simulink model "SIMULINK_U_a_C"  (R2023b)
settings: Solver=FixedStepAuto  StartTime=0.0  StopTime=sim_end_time  FixedStep=fixed_step_size  RelTol=1e-3
undefined symbols (not defined in the file): a, act_end, b, battery_threshold, bb, draw_gif, droneyeeUAV2_NUM, droneyeeUAV3_NUM, droneyeeUAV4_NUM, droneyeeUAV5_NUM, fixed_step_size, k, KD_x, KD_y, kd_z, KDD_x, KDD_y, KI_x, KI_y, ki_z, KII_x, KII_y, KP_x, KP_y, kp_z, KPP_x, KPP_y, lmt, omega, R, sim_end_time, uav10num, uav1num, uav2num, uav3num, uav4num, uav5num, uav6num, uav7num, uav8num, uav9num, UAV_NUM, Vel_Switch_1, Vel_Switch_10, Vel_Switch_11, Vel_Switch_12, Vel_Switch_13, Vel_Switch_14, Vel_Switch_15, Vel_Switch_16, Vel_Switch_17, Vel_Switch_18, Vel_Switch_19, Vel_Switch_2, Vel_Switch_20, Vel_Switch_3, Vel_Switch_4, Vel_Switch_5, Vel_Switch_6, Vel_Switch_7 ... (+11)
libraries: simulink x120, aerolibanimutils x1
(part 4 of 10)

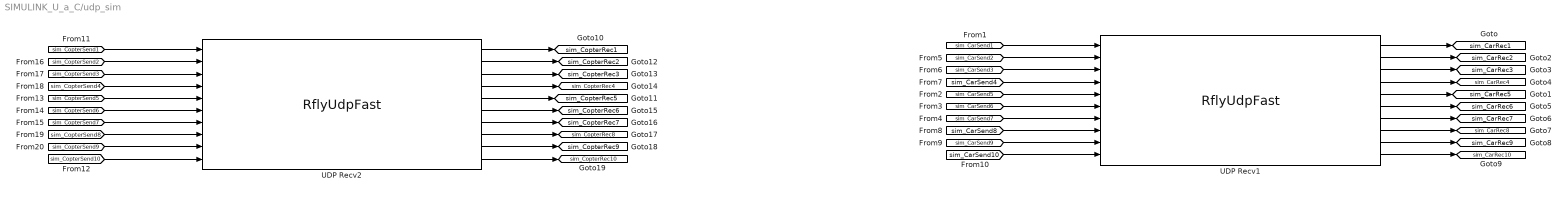
== system SIMULINK_U_a_C/udp_sim ==
  UDP Recv1 : S-Function  FunctionName=RflyUdpFast  Parameters=port,num,modeValue,T,ip  SFunctionDeploymentMode=off  EnableBusSupport=off  mask(UDP Receive){ip=127.0.0.1, port=20100, num=10, mode=UltraSimple Mode, T=1/30, modeValue=0}
      mask prompts: ip "UDP IP Address"; port "UDP Port"; num "vehicle Number"; mode "UDP Mode"; T "Sample Time"
      mask help:
      | This block receives bytes from an UDP/IP connection.
      | The first parameter is the UDP port on the first CopterSim App
      | The second parameter is the total vehicle number
      | The third parameter is the data mode. check the help button for the definition
      mask init:
      | if strcmp(mode,'FullData Mode')
      |     modeValue = 0;
      | elseif strcmp(mode,'SimpleData Mode') 
      |     modeValue = 1;
      | elseif strcmp(mode,'UltraSimple Mode') 
      |     modeValue = 2;
      | else
      |     modeValue = 0;
      | end
      mask Help:
      | UDP mode = 0 (localhost) or 1(broadcast), the 28-D output is defined as:
      | for(int i=0;i<3;i++){
      |     data[0+i]=(double)stl.gpsHome[i];
      |     data[3+i]=(double)stl.AngEular[i];
      |     data[6+i]=(double)stl.localPos[i];
      |     data[9+i]=(double)stl.localVel[i];
      |     data[12+i]=(double)stl.GpsPos[i];
      |     data[15+i]=(double)stl.GpsVel[i];
      | }
      | data[18] = (double)stl.time_boot_ms;
      | data[19] = (double)stl.copterID;
      | data[20] = (double)stl.relative_alt;
      | data[21] = (double)stl.hdg;
      | data[22] = (double)stl.satellites_visible;
      | data[23] = (double)stl.fix_type;
      | data[24] = (double)stl.resrveInit;
      | data[25] = (double)stl.pos_horiz_accuracy;
      | data[26] = (double)stl.pos_vert_accuracy;
      | data[27] = (double)stl.resrveFloat;
      | 
      | UDP mode =  2 (localhost) or 3(broadcast), 4,5 the 12-D output is defined as:
      | 
      | if(iUdpMode==2||iUdpMode==3){
      |     for(int i=0;i<3;i++){
      |         data[i]=(double)st.gpsHome[i];
      |         data[i+3]=(double)st.AngEular[i];
      |         data[i+6]=(double)st.localPos[i];
      |         data[i+9]=(double)st.localVel[i];
      |     }
      | }
      | if(iUdpMode==4||iUdpMode==5){
      |     double GpsHomePos[3];
      |     for(int i=0;i<3;i++){
      |             GpsHomePos[i] = (double)st.gpsHome[i];
      |             data[3+i]=(double)st.localPos[i];
      |             data[6+i]=(double)st.localVel[i];
      |             data[9+i]=(double)st.AngEular[i];
      |     }
      |     double PIR = 3.1415926536;
      |     data[0]=(GpsHomePos[0]*1e-7-40.1540302)/180*PIR*6362000+(double)st.localPos[0];
      |     data[1]=(GpsHomePos[1]*1e-7-116.2593683)/180*PIR*6362000+(double)st.localPos[1];
      |     data[2]=-GpsHomePos[2]*1e-3+(double)st.localPos[2];
      | }
      | 
      | The above structure is
      | struct outHILStateData{ // mavlink data forward from Pixhawk
      |     uint32_t time_boot_ms; //Timestamp of the message
      |     uint32_t copterID;     //Copter ID start from 1
      |     int32_t GpsPos[3];     //Estimated GPS position，lat&long: deg*1e7, alt: m*1e3 and up is positive
      |     int32_t GpsVel[3];     //Estimated GPS velocity, NED, m/s*1e2->cm/s
      |     int32_t gpsHome[3];     //Home GPS position, lat&long: deg*1e7, alt: m*1e3 and up is positive
      |     int32_t relative_alt;  //alt: m*1e3 and up is positive
      |     int32_t hdg;           //Course angle, NED,deg*1000, 0~360
      |     int32_t satellites_visible; //GPS Raw data, sum of satellite
      |     int32_t fix_type;     //GPS Raw data, Fixed type, 3 for fixed (good precision)
      |     int32_t resrveInit;       //Int, reserve for the future use
      |     float AngEular[3];    //Estimated Euler angle, unit: rad/s
      |     float localPos[3];    //Estimated locoal position, NED, unit: m
      |     float localVel[3];    //Estimated locoal velocity, NED, unit: m/s
      |     float pos_horiz_accuracy;   //GPS horizontal accuracy, unit: m
      |     float pos_vert_accuracy; //GPS vertical accuracy, unit: m
      |     float resrveFloat;      //float,reserve for the future use
      | }
      mask TypeOptions mode: FullData Mode | SimpleData Mode | UltraSimple Mode
  UDP Recv2 : S-Function  FunctionName=RflyUdpFast  Parameters=port,num,modeValue,T,ip  SFunctionDeploymentMode=off  EnableBusSupport=off  mask(UDP Receive){ip=127.0.0.1, port=20100, num=10, mode=UltraSimple Mode, T=1/30, modeValue=0}
      mask prompts: ip "UDP IP Address"; port "UDP Port"; num "vehicle Number"; mode "UDP Mode"; T "Sample Time"
      mask help:
      | This block receives bytes from an UDP/IP connection.
      | The first parameter is the UDP port on the first CopterSim App
      | The second parameter is the total vehicle number
      | The third parameter is the data mode. check the help button for the definition
      mask init:
      | if strcmp(mode,'FullData Mode')
      |     modeValue = 0;
      | elseif strcmp(mode,'SimpleData Mode') 
      |     modeValue = 1;
      | elseif strcmp(mode,'UltraSimple Mode') 
      |     modeValue = 2;
      | else
      |     modeValue = 0;
      | end
      mask Help:
      | UDP mode = 0 (localhost) or 1(broadcast), the 28-D output is defined as:
      | for(int i=0;i<3;i++){
      |     data[0+i]=(double)stl.gpsHome[i];
      |     data[3+i]=(double)stl.AngEular[i];
      |     data[6+i]=(double)stl.localPos[i];
      |     data[9+i]=(double)stl.localVel[i];
      |     data[12+i]=(double)stl.GpsPos[i];
      |     data[15+i]=(double)stl.GpsVel[i];
      | }
      | data[18] = (double)stl.time_boot_ms;
      | data[19] = (double)stl.copterID;
      | data[20] = (double)stl.relative_alt;
      | data[21] = (double)stl.hdg;
      | data[22] = (double)stl.satellites_visible;
      | data[23] = (double)stl.fix_type;
      | data[24] = (double)stl.resrveInit;
      | data[25] = (double)stl.pos_horiz_accuracy;
      | data[26] = (double)stl.pos_vert_accuracy;
      | data[27] = (double)stl.resrveFloat;
      | 
      | UDP mode =  2 (localhost) or 3(broadcast), 4,5 the 12-D output is defined as:
      | 
      | if(iUdpMode==2||iUdpMode==3){
      |     for(int i=0;i<3;i++){
      |         data[i]=(double)st.gpsHome[i];
      |         data[i+3]=(double)st.AngEular[i];
      |         data[i+6]=(double)st.localPos[i];
      |         data[i+9]=(double)st.localVel[i];
      |     }
      | }
      | if(iUdpMode==4||iUdpMode==5){
      |     double GpsHomePos[3];
      |     for(int i=0;i<3;i++){
      |             GpsHomePos[i] = (double)st.gpsHome[i];
      |             data[3+i]=(double)st.localPos[i];
      |             data[6+i]=(double)st.localVel[i];
      |             data[9+i]=(double)st.AngEular[i];
      |     }
      |     double PIR = 3.1415926536;
      |     data[0]=(GpsHomePos[0]*1e-7-40.1540302)/180*PIR*6362000+(double)st.localPos[0];
      |     data[1]=(GpsHomePos[1]*1e-7-116.2593683)/180*PIR*6362000+(double)st.localPos[1];
      |     data[2]=-GpsHomePos[2]*1e-3+(double)st.localPos[2];
      | }
      | 
      | The above structure is
      | struct outHILStateData{ // mavlink data forward from Pixhawk
      |     uint32_t time_boot_ms; //Timestamp of the message
      |     uint32_t copterID;     //Copter ID start from 1
      |     int32_t GpsPos[3];     //Estimated GPS position，lat&long: deg*1e7, alt: m*1e3 and up is positive
      |     int32_t GpsVel[3];     //Estimated GPS velocity, NED, m/s*1e2->cm/s
      |     int32_t gpsHome[3];     //Home GPS position, lat&long: deg*1e7, alt: m*1e3 and up is positive
      |     int32_t relative_alt;  //alt: m*1e3 and up is positive
      |     int32_t hdg;           //Course angle, NED,deg*1000, 0~360
      |     int32_t satellites_visible; //GPS Raw data, sum of satellite
      |     int32_t fix_type;     //GPS Raw data, Fixed type, 3 for fixed (good precision)
      |     int32_t resrveInit;       //Int, reserve for the future use
      |     float AngEular[3];    //Estimated Euler angle, unit: rad/s
      |     float localPos[3];    //Estimated locoal position, NED, unit: m
      |     float localVel[3];    //Estimated locoal velocity, NED, unit: m/s
      |     float pos_horiz_accuracy;   //GPS horizontal accuracy, unit: m
      |     float pos_vert_accuracy; //GPS vertical accuracy, unit: m
      |     float resrveFloat;      //float,reserve for the future use
      | }
      mask TypeOptions mode: FullData Mode | SimpleData Mode | UltraSimple Mode
  tag scope: sim_CarRec10=global, sim_CarRec1=global, sim_CarRec2=global, sim_CarRec3=global, sim_CarRec4=global, sim_CarRec5=global, sim_CarRec6=global, sim_CarRec7=global, sim_CarRec8=global, sim_CarRec9=global, sim_CopterRec10=global, sim_CopterRec1=global, sim_CopterRec2=global, sim_CopterRec3=global, sim_CopterRec4=global, sim_CopterRec5=global, sim_CopterRec6=global, sim_CopterRec7=global, sim_CopterRec8=global, sim_CopterRec9=global
  wires:
  UDP Recv1/9 -> [sim_CarRec9]
  UDP Recv1/8 -> [sim_CarRec8]
  [sim_CarSend10] -> UDP Recv1/10
  [sim_CarSend3] -> UDP Recv1/3
  [sim_CarSend5] -> UDP Recv1/5
  [sim_CarSend9] -> UDP Recv1/9
  [sim_CarSend6] -> UDP Recv1/6
  UDP Recv1/1 -> [sim_CarRec1]
  [sim_CarSend8] -> UDP Recv1/8
  UDP Recv1/7 -> [sim_CarRec7]
  UDP Recv1/5 -> [sim_CarRec5]
  UDP Recv1/2 -> [sim_CarRec2]
  [sim_CarSend7] -> UDP Recv1/7
  [sim_CarSend4] -> UDP Recv1/4
  UDP Recv1/4 -> [sim_CarRec4]
  UDP Recv1/10 -> [sim_CarRec10]
  [sim_CarSend2] -> UDP Recv1/2
  UDP Recv1/6 -> [sim_CarRec6]
  [sim_CarSend1] -> UDP Recv1/1
  UDP Recv1/3 -> [sim_CarRec3]
  [sim_CopterSend3] -> UDP Recv2/3
  UDP Recv2/5 -> [sim_CopterRec5]
  UDP Recv2/7 -> [sim_CopterRec7]
  UDP Recv2/6 -> [sim_CopterRec6]
  UDP Recv2/1 -> [sim_CopterRec1]
  [sim_CopterSend7] -> UDP Recv2/7
  [sim_CopterSend2] -> UDP Recv2/2
  [sim_CopterSend10] -> UDP Recv2/10
  UDP Recv2/9 -> [sim_CopterRec9]
  [sim_CopterSend8] -> UDP Recv2/8
  UDP Recv2/2 -> [sim_CopterRec2]
  UDP Recv2/10 -> [sim_CopterRec10]
  UDP Recv2/8 -> [sim_CopterRec8]
  UDP Recv2/3 -> [sim_CopterRec3]
  [sim_CopterSend9] -> UDP Recv2/9
  [sim_CopterSend4] -> UDP Recv2/4
  [sim_CopterSend6] -> UDP Recv2/6
  [sim_CopterSend1] -> UDP Recv2/1
  [sim_CopterSend5] -> UDP Recv2/5
  UDP Recv2/4 -> [sim_CopterRec4]

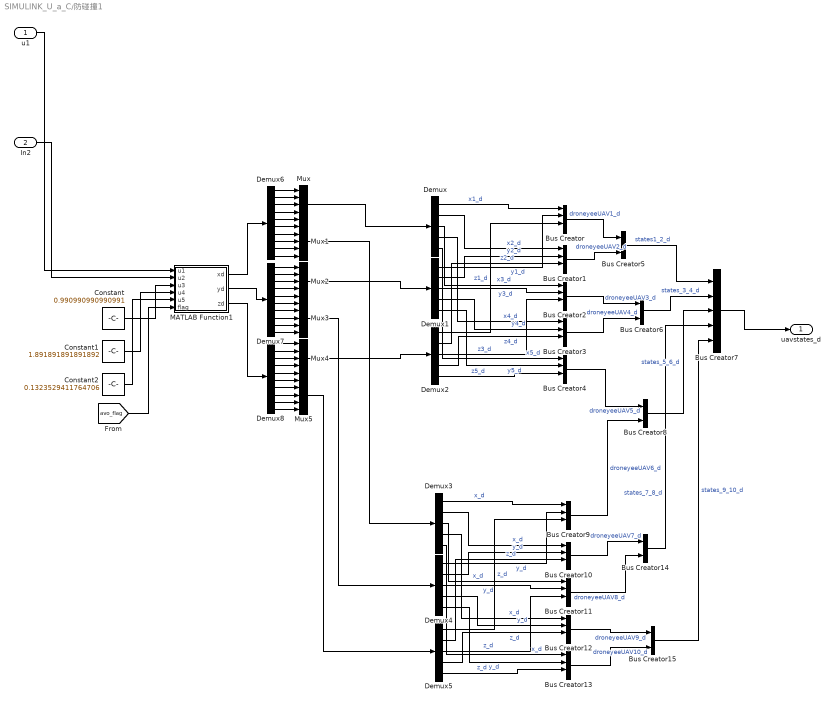
== system SIMULINK_U_a_C/防碰撞1 ==
  u1 : Inport
  In2 : Inport  Port=2
  Bus Creator{,1..4,9..13} (10 alike) : BusCreator  Inputs=4
  Bus Creator{5..6,8,14..15} (5 alike) : BusCreator  Inputs=2
  Bus Creator7 : BusCreator  Inputs=5
  Constant : Constant  Value=0.990990990990991
  Constant1 : Constant  Value=1.891891891891892
  Constant2 : Constant  Value=0.1323529411764706
  Demux{,1..5} (6 alike) : Demux  Outputs=5
  Demux6 : Demux  Outputs=10
  Demux7 : Demux  Outputs=10
  Demux8 : Demux  Outputs=10
  MATLAB Function1 : MATLAB Function
  Mux{,1..5} (6 alike) : Mux  Inputs=5
  uavstates_d : Outport  VectorParamsAs1DForOutWhenUnconnected=off
  wires:
  Bus Creator3/1 -> Bus Creator6/2  "droneyeeUAV4_d"
  Bus Creator1/1 -> Bus Creator5/2  "droneyeeUAV2_d"
  Bus Creator2/1 -> Bus Creator6/1  "droneyeeUAV3_d"
  Demux1/2 -> Bus Creator1/2  "y2_d"
  Bus Creator/1 -> Bus Creator5/1  "droneyeeUAV1_d"
  Bus Creator4/1 -> Bus Creator8/1  "droneyeeUAV5_d"
  Bus Creator6/1 -> Bus Creator7/2  "states_3_4_d"
  Bus Creator5/1 -> Bus Creator7/1  "states1_2_d"
  In2/1 -> MATLAB Function1/2(u2)
  u1/1 -> MATLAB Function1/1(u1)
  Demux2/2 -> Bus Creator1/3  "z2_d"
  Demux2/4 -> Bus Creator3/3  "z4_d"
  Demux/3 -> Bus Creator2/1  "x3_d"
  Demux2/5 -> Bus Creator4/3  "z5_d"
  Demux1/4 -> Bus Creator3/2  "y4_d"
  MATLAB Function1/3(zd) -> Demux8/1
  MATLAB Function1/2(yd) -> Demux7/1
  Demux1/5 -> Bus Creator4/2  "y5_d"
  Demux1/3 -> Bus Creator2/2  "y3_d"
  Demux2/3 -> Bus Creator2/3  "z3_d"
  Demux/4 -> Bus Creator3/1  "x4_d"
  Demux/5 -> Bus Creator4/1  "x5_d"
  Demux/1 -> Bus Creator/1  "x1_d"
  Demux/2 -> Bus Creator1/1  "x2_d"
  Demux1/1 -> Bus Creator/2  "y1_d"
  Demux2/1 -> Bus Creator/3  "z1_d"
  MATLAB Function1/1(xd) -> Demux6/1
  Bus Creator7/1 -> uavstates_d/1
  ? -> Bus Creator/4  "yaw1_d"
  ? -> Bus Creator1/4  "yaw2_d"
  ? -> Bus Creator2/4  "yaw3_d"
  ? -> Bus Creator3/4  "yaw4_d"
  ? -> Bus Creator4/4  "yaw5_d"
  Constant/1 -> MATLAB Function1/3(u3)
  Constant1/1 -> MATLAB Function1/4(u4)
  Constant2/1 -> MATLAB Function1/5(u5)
  ? -> Bus Creator13/4  "yaw_d"
  ? -> Bus Creator11/4  "yaw_d"
  ? -> Bus Creator10/4  "yaw_d"
  ? -> Bus Creator9/4  "yaw_d"
  ? -> Bus Creator12/4  "yaw_d"
  Demux5/2 -> Bus Creator10/3  "z_d"
  Demux3/2 -> Bus Creator10/1  "x_d"
  Demux5/5 -> Bus Creator13/3  "z_d"
  Demux3/4 -> Bus Creator12/1  "x_d"
  Demux3/1 -> Bus Creator9/1  "x_d"
  Demux5/4 -> Bus Creator12/3  "z_d"
  Demux5/1 -> Bus Creator9/3  "z_d"
  Demux5/3 -> Bus Creator11/3  "z_d"
  Demux4/1 -> Bus Creator9/2  "y_d"
  Demux4/3 -> Bus Creator11/2  "y_d"
  Demux3/5 -> Bus Creator13/1  "x_d"
  Demux3/3 -> Bus Creator11/1  "x_d"
  Demux4/4 -> Bus Creator12/2  "y_d"
  Demux4/2 -> Bus Creator10/2  "y_d"
  Demux4/5 -> Bus Creator13/2  "y_d"
  Demux6/1 -> Mux/1
  Demux6/2 -> Mux/2
  Demux6/3 -> Mux/3
  Demux6/4 -> Mux/4
  Demux6/5 -> Mux/5
  Demux6/6 -> Mux1/1
  Demux6/7 -> Mux1/2
  Demux6/8 -> Mux1/3
  Demux6/9 -> Mux1/4
  Demux6/10 -> Mux1/5
  Demux7/6 -> Mux3/1
  Demux7/10 -> Mux3/5
  Demux7/8 -> Mux3/3
  Demux7/4 -> Mux2/4
  Demux7/3 -> Mux2/3
  Demux7/5 -> Mux2/5
  Demux7/7 -> Mux3/2
  Demux7/2 -> Mux2/2
  Demux7/9 -> Mux3/4
  Demux7/1 -> Mux2/1
  Demux8/6 -> Mux5/1
  Demux8/10 -> Mux5/5
  Demux8/8 -> Mux5/3
  Demux8/4 -> Mux4/4
  Demux8/3 -> Mux4/3
  Demux8/5 -> Mux4/5
  Demux8/7 -> Mux5/2
  Demux8/2 -> Mux4/2
  Demux8/9 -> Mux5/4
  Demux8/1 -> Mux4/1
  Mux/1 -> Demux/1
  Mux1/1 -> Demux3/1
  Mux2/1 -> Demux1/1
  Mux3/1 -> Demux4/1
  Mux4/1 -> Demux2/1
  Mux5/1 -> Demux5/1
  [avo_flag] -> MATLAB Function1/6(flag)
  Bus Creator9/1 -> Bus Creator8/2  "droneyeeUAV6_d"
  Bus Creator8/1 -> Bus Creator7/3  "states_5_6_d"
  Bus Creator10/1 -> Bus Creator14/1  "droneyeeUAV7_d"
  Bus Creator11/1 -> Bus Creator14/2  "droneyeeUAV8_d"
  Bus Creator12/1 -> Bus Creator15/1  "droneyeeUAV9_d"
  Bus Creator13/1 -> Bus Creator15/2  "droneyeeUAV10_d"
  Bus Creator14/1 -> Bus Creator7/4  "states_7_8_d"
  Bus Creator15/1 -> Bus Creator7/5  "states_9_10_d"

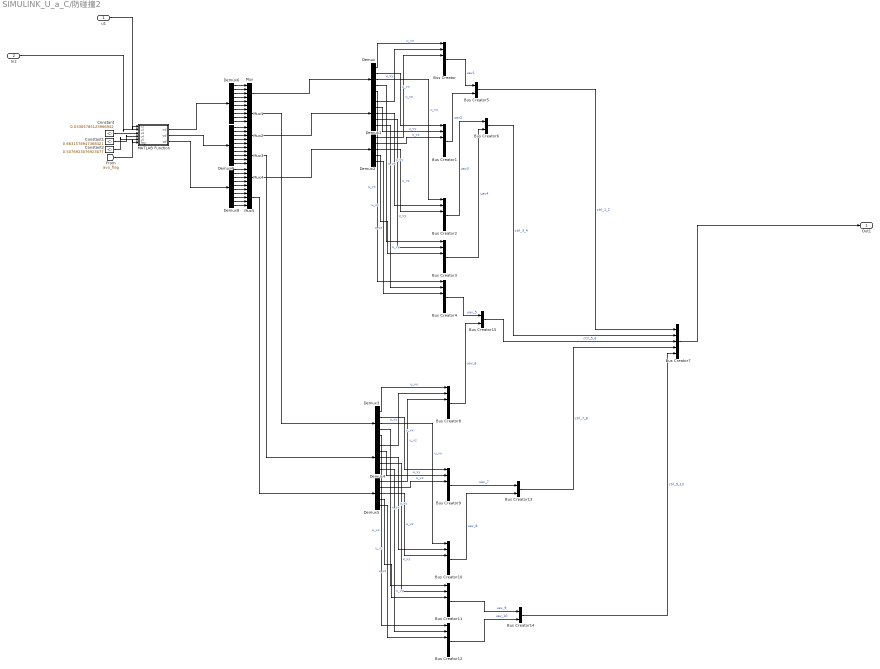
== system SIMULINK_U_a_C/防碰撞2 ==
  u1 : Inport
  In2 : Inport  Port=2
  Bus Creator{,1..4,8..12} (10 alike) : BusCreator  Inputs=6
  Bus Creator{5..6,13..15} (5 alike) : BusCreator  Inputs=2
  Bus Creator7 : BusCreator  Inputs=5
  Constant : Constant  Value=0.03305785123966942
  Constant1 : Constant  Value=0.6631578947368421
  Constant2 : Constant  Value=0.5076923076923077
  Demux{,1..5} (6 alike) : Demux  Outputs=5
  Demux6 : Demux  Outputs=10
  Demux7 : Demux  Outputs=10
  Demux8 : Demux  Outputs=10
  MATLAB Function : MATLAB Function
  Mux{,1..5} (6 alike) : Mux  Inputs=5
  Out1 : Outport  VectorParamsAs1DForOutWhenUnconnected=off
  wires:
  Bus Creator3/1 -> Bus Creator6/2  "uav4"
  Bus Creator1/1 -> Bus Creator5/2  "uav2"
  Bus Creator2/1 -> Bus Creator6/1  "uav3"
  Bus Creator/1 -> Bus Creator5/1  "uav1"
  Bus Creator15/1 -> Bus Creator7/3  "ctrl_5_6"
  Bus Creator6/1 -> Bus Creator7/2  "ctrl_3_4"
  Bus Creator5/1 -> Bus Creator7/1  "ctrl_1_2"
  In2/1 -> MATLAB Function/2(u2)
  u1/1 -> MATLAB Function/1(u1)
  MATLAB Function/3(zd) -> Demux8/1
  MATLAB Function/2(yd) -> Demux7/1
  Demux/1 -> Bus Creator/1  "u_vx"
  Demux1/1 -> Bus Creator/2  "u_vy"
  Demux2/1 -> Bus Creator/3  "u_vz"
  MATLAB Function/1(xd) -> Demux6/1
  Bus Creator7/1 -> Out1/1
  ? -> Bus Creator/4  "u_rate_roll"
  ? -> Bus Creator/5  "u_rate_pitch"
  ? -> Bus Creator/6  "u_rate_yaw"
  ? -> Bus Creator4/6  "u_rate_yaw"
  ? -> Bus Creator4/4  "u_rate_roll"
  Demux2/5 -> Bus Creator4/3  "u_vz"
  Demux/5 -> Bus Creator4/1  "u_vx"
  Demux1/5 -> Bus Creator4/2  "u_vy"
  ? -> Bus Creator4/5  "u_rate_pitch"
  ? -> Bus Creator3/6  "u_rate_yaw"
  ? -> Bus Creator3/4  "u_rate_roll"
  Demux2/4 -> Bus Creator3/3  "u_vz"
  Demux/4 -> Bus Creator3/1  "u_vx"
  Demux1/4 -> Bus Creator3/2  "u_vy"
  ? -> Bus Creator3/5  "u_rate_pitch"
  ? -> Bus Creator2/6  "u_rate_yaw"
  ? -> Bus Creator2/4  "u_rate_roll"
  Demux2/3 -> Bus Creator2/3  "u_vz"
  Demux/3 -> Bus Creator2/1  "u_vx"
  Demux1/3 -> Bus Creator2/2  "u_vy"
  ? -> Bus Creator2/5  "u_rate_pitch"
  ? -> Bus Creator1/6  "u_rate_yaw"
  ? -> Bus Creator1/4  "u_rate_roll"
  Demux2/2 -> Bus Creator1/3  "u_vz"
  Demux/2 -> Bus Creator1/1  "u_vx"
  Demux1/2 -> Bus Creator1/2  "u_vy"
  ? -> Bus Creator1/5  "u_rate_pitch"
  Constant/1 -> MATLAB Function/3(u3)
  Constant1/1 -> MATLAB Function/4(u4)
  Constant2/1 -> MATLAB Function/5(u5)
  Demux3/1 -> Bus Creator8/1  "u_vx"
  Demux5/3 -> Bus Creator10/3  "u_vz"
  Demux4/4 -> Bus Creator11/2  "u_vy"
  ? -> Bus Creator10/4  "u_rate_roll"
  ? -> Bus Creator10/5  "u_rate_pitch"
  ? -> Bus Creator9/5  "u_rate_pitch"
  Demux5/1 -> Bus Creator8/3  "u_vz"
  Demux3/2 -> Bus Creator9/1  "u_vx"
  Demux4/2 -> Bus Creator9/2  "u_vy"
  Demux3/5 -> Bus Creator12/1  "u_vx"
  Bus Creator10/1 -> Bus Creator13/2  "uav_8"
  Demux4/5 -> Bus Creator12/2  "u_vy"
  Demux3/4 -> Bus Creator11/1  "u_vx"
  Demux3/3 -> Bus Creator10/1  "u_vx"
  ? -> Bus Creator10/6  "u_rate_yaw"
  Demux5/4 -> Bus Creator11/3  "u_vz"
  ? -> Bus Creator9/6  "u_rate_yaw"
  Demux5/2 -> Bus Creator9/3  "u_vz"
  Demux4/3 -> Bus Creator10/2  "u_vy"
  ? -> Bus Creator12/5  "u_rate_pitch"
  ? -> Bus Creator9/4  "u_rate_roll"
  ? -> Bus Creator12/6  "u_rate_yaw"
  ? -> Bus Creator8/6  "u_rate_yaw"
  ? -> Bus Creator11/6  "u_rate_yaw"
  ? -> Bus Creator8/4  "u_rate_roll"
  ? -> Bus Creator11/4  "u_rate_roll"
  Bus Creator9/1 -> Bus Creator13/1  "uav_7"
  Bus Creator11/1 -> Bus Creator14/1  "uav_9"
  ? -> Bus Creator8/5  "u_rate_pitch"
  Bus Creator8/1 -> Bus Creator15/2  "uav_6"
  Demux4/1 -> Bus Creator8/2  "u_vy"
  ? -> Bus Creator11/5  "u_rate_pitch"
  ? -> Bus Creator12/4  "u_rate_roll"
  Demux5/5 -> Bus Creator12/3  "u_vz"
  Demux6/4 -> Mux/4
  Demux6/3 -> Mux/3
  Demux6/2 -> Mux/2
  Demux8/7 -> Mux5/2
  Demux7/8 -> Mux3/3
  Demux8/10 -> Mux5/5
  Demux7/6 -> Mux3/1
  Demux6/8 -> Mux1/3
  Demux6/6 -> Mux1/1
  Demux7/1 -> Mux2/1
  Demux7/4 -> Mux2/4
  Demux7/2 -> Mux2/2
  Demux7/7 -> Mux3/2
  Demux7/9 -> Mux3/4
  Demux7/5 -> Mux2/5
  Demux6/7 -> Mux1/2
  Demux6/5 -> Mux/5
  Demux6/10 -> Mux1/5
  Demux8/2 -> Mux4/2
  Demux8/4 -> Mux4/4
  Demux6/9 -> Mux1/4
  Demux8/6 -> Mux5/1
  Demux7/10 -> Mux3/5
  Demux7/3 -> Mux2/3
  Demux8/9 -> Mux5/4
  Demux8/1 -> Mux4/1
  Demux6/1 -> Mux/1
  Demux8/8 -> Mux5/3
  Demux8/3 -> Mux4/3
  Demux8/5 -> Mux4/5
  Mux/1 -> Demux/1
  Mux2/1 -> Demux1/1
  Mux4/1 -> Demux2/1
  Mux1/1 -> Demux3/1
  Mux3/1 -> Demux4/1
  Mux5/1 -> Demux5/1
  [avo_flag] -> MATLAB Function/6(flag)
  Bus Creator4/1 -> Bus Creator15/1  "uav_5"
  Bus Creator12/1 -> Bus Creator14/2  "uav_10"
  Bus Creator13/1 -> Bus Creator7/4  "ctrl_7_8"
  Bus Creator14/1 -> Bus Creator7/5  "ctrl_9_10"

== system SIMULINK_U_a_C/CMD_UAV/CMD1 ==
  "clock " : Inport
  droneyeeUAV_states : Inport  Port=2
  droneyeeUAV_bat : Inport  Port=3
  Bus Selector : BusSelector  OutputSignals=x,y,z
  Constant : Constant  Value=sim_end_time
  Constant1 : Constant  Value=battery_threshold
  Constant2 : Constant  Value=z_d_for_land
  Constant3 : Constant  Value=0
  Constant4 : Constant  Value=UAV_NUM
  MATLAB Function1 : MATLAB Function  TreatAsAtomicUnit=on
  Manual Switch2 : ManualSwitch
  Sine Wave2 : Sin  Amplitude=0.3  Frequency=1.0
  Slider Gain3 : simulink/Math Operations/Slider Gain  gain=1  low=0  high=2
  Subsystem : Subsystem
  x_d : Outport  VectorParamsAs1DForOutWhenUnconnected=off
  y_d : Outport  Port=2  VectorParamsAs1DForOutWhenUnconnected=off
  z_d : Outport  Port=3  VectorParamsAs1DForOutWhenUnconnected=off
  yaw_d : Outport  Port=4  VectorParamsAs1DForOutWhenUnconnected=off
  wires:
  Manual Switch2/1 -> Slider Gain3/1
  Slider Gain3/1 -> yaw_d/1
  Sine Wave2/1 -> Manual Switch2/2
  Constant3/1 -> Manual Switch2/1
  MATLAB Function1/2(y_d_) -> y_d/1
  Constant2/1 -> MATLAB Function1/11(z_d_for_land)
  Subsystem/3(zd) -> MATLAB Function1/3(z_d)
  Constant1/1 -> MATLAB Function1/10(battery_threshold)
  MATLAB Function1/3(z_d_) -> z_d/1
  droneyeeUAV_states/1 -> Subsystem/2(uavstates), Bus Selector/1
  MATLAB Function1/1(x_d_) -> x_d/1
  Constant4/1 -> MATLAB Function1/12(UAV_NUM)
  Constant/1 -> MATLAB Function1/9(sim_time_end)
  Subsystem/1("xd ") -> MATLAB Function1/1(x_d)
  Subsystem/2(yd) -> MATLAB Function1/2(y_d)
  "clock "/1 -> Subsystem/1(clock), MATLAB Function1/4(timestamp)
  droneyeeUAV_bat/1 -> MATLAB Function1/8(battery_status)
  Bus Selector/1 -> MATLAB Function1/5(x)  "<x>"
  Bus Selector/2 -> MATLAB Function1/6(y)  "<y>"
  Bus Selector/3 -> MATLAB Function1/7(z)  "<z>"

== system SIMULINK_U_a_C/CMD_UAV/CMD10 ==
  "clock " : Inport
  droneyeeUAV_states : Inport  Port=2
  droneyeeUAV_bat : Inport  Port=3
  Bus Selector : BusSelector  OutputSignals=x,y,z
  Constant : Constant  Value=sim_end_time
  Constant1 : Constant  Value=battery_threshold
  Constant2 : Constant  Value=z_d_for_land
  Constant3 : Constant  Value=0
  Constant4 : Constant  Value=UAV_NUM
  MATLAB Function1 : MATLAB Function  TreatAsAtomicUnit=on
  Manual Switch2 : ManualSwitch
  Sine Wave2 : Sin  Amplitude=0.3  Frequency=1.0
  Slider Gain3 : simulink/Math Operations/Slider Gain  gain=1  low=0  high=2
  Subsystem : Subsystem
  x_d : Outport  VectorParamsAs1DForOutWhenUnconnected=off
  y_d : Outport  Port=2  VectorParamsAs1DForOutWhenUnconnected=off
  z_d : Outport  Port=3  VectorParamsAs1DForOutWhenUnconnected=off
  yaw_d : Outport  Port=4  VectorParamsAs1DForOutWhenUnconnected=off
  wires:
  Manual Switch2/1 -> Slider Gain3/1
  Slider Gain3/1 -> yaw_d/1
  Sine Wave2/1 -> Manual Switch2/2
  Constant3/1 -> Manual Switch2/1
  MATLAB Function1/2(y_d_) -> y_d/1
  Constant2/1 -> MATLAB Function1/11(z_d_for_land)
  Subsystem/3(zd) -> MATLAB Function1/3(z_d)
  Constant1/1 -> MATLAB Function1/10(battery_threshold)
  MATLAB Function1/3(z_d_) -> z_d/1
  droneyeeUAV_states/1 -> Subsystem/2(uavstates), Bus Selector/1
  MATLAB Function1/1(x_d_) -> x_d/1
  Constant4/1 -> MATLAB Function1/12(UAV_NUM)
  Constant/1 -> MATLAB Function1/9(sim_time_end)
  Subsystem/1("xd ") -> MATLAB Function1/1(x_d)
  Subsystem/2(yd) -> MATLAB Function1/2(y_d)
  "clock "/1 -> Subsystem/1(clock), MATLAB Function1/4(timestamp)
  droneyeeUAV_bat/1 -> MATLAB Function1/8(battery_status)
  Bus Selector/1 -> MATLAB Function1/5(x)  "<x>"
  Bus Selector/2 -> MATLAB Function1/6(y)  "<y>"
  Bus Selector/3 -> MATLAB Function1/7(z)  "<z>"

== system SIMULINK_U_a_C/CMD_UAV/CMD2 ==
  "clock " : Inport
  droneyeeUAV_states : Inport  Port=2
  droneyeeUAV_bat : Inport  Port=3
  Bus Selector : BusSelector  OutputSignals=x,y,z
  Constant : Constant  Value=sim_end_time
  Constant1 : Constant  Value=battery_threshold
  Constant2 : Constant  Value=z_d_for_land
  Constant3 : Constant  Value=0
  Constant4 : Constant  Value=UAV_NUM
  MATLAB Function1 : MATLAB Function  TreatAsAtomicUnit=on
  Manual Switch2 : ManualSwitch
  Sine Wave2 : Sin  Amplitude=0.3  Frequency=1.0
  Slider Gain3 : simulink/Math Operations/Slider Gain  gain=1  low=0  high=2
  Subsystem : Subsystem
  x_d : Outport  VectorParamsAs1DForOutWhenUnconnected=off
  y_d : Outport  Port=2  VectorParamsAs1DForOutWhenUnconnected=off
  z_d : Outport  Port=3  VectorParamsAs1DForOutWhenUnconnected=off
  yaw_d : Outport  Port=4  VectorParamsAs1DForOutWhenUnconnected=off
  wires:
  Manual Switch2/1 -> Slider Gain3/1
  Slider Gain3/1 -> yaw_d/1
  Sine Wave2/1 -> Manual Switch2/2
  Constant3/1 -> Manual Switch2/1
  Bus Selector/1 -> MATLAB Function1/5(x)  "<x>"
  MATLAB Function1/2(y_d_) -> y_d/1
  Constant2/1 -> MATLAB Function1/11(z_d_for_land)
  Subsystem/3(zd) -> MATLAB Function1/3(z_d)
  Bus Selector/2 -> MATLAB Function1/6(y)  "<y>"
  Constant1/1 -> MATLAB Function1/10(battery_threshold)
  MATLAB Function1/3(z_d_) -> z_d/1
  droneyeeUAV_states/1 -> Subsystem/2(uavstates), Bus Selector/1
  MATLAB Function1/1(x_d_) -> x_d/1
  Constant4/1 -> MATLAB Function1/12(UAV_NUM)
  Bus Selector/3 -> MATLAB Function1/7(z)  "<z>"
  Constant/1 -> MATLAB Function1/9(sim_time_end)
  Subsystem/1("xd ") -> MATLAB Function1/1(x_d)
  Subsystem/2(yd) -> MATLAB Function1/2(y_d)
  "clock "/1 -> Subsystem/1(clock), MATLAB Function1/4(timestamp)
  droneyeeUAV_bat/1 -> MATLAB Function1/8(battery_status)

== system SIMULINK_U_a_C/CMD_UAV/CMD3 ==
  "clock " : Inport
  droneyeeUAV_states : Inport  Port=2
  droneyeeUAV_bat : Inport  Port=3
  Bus Selector : BusSelector  OutputSignals=x,y,z
  Constant : Constant  Value=sim_end_time
  Constant1 : Constant  Value=battery_threshold
  Constant2 : Constant  Value=z_d_for_land
  Constant3 : Constant  Value=0
  Constant4 : Constant  Value=UAV_NUM
  MATLAB Function1 : MATLAB Function  TreatAsAtomicUnit=on
  Manual Switch2 : ManualSwitch
  Sine Wave2 : Sin  Amplitude=0.3  Frequency=1.0
  Slider Gain3 : simulink/Math Operations/Slider Gain  gain=1  low=0  high=2
  Subsystem : Subsystem
  x_d : Outport  VectorParamsAs1DForOutWhenUnconnected=off
  y_d : Outport  Port=2  VectorParamsAs1DForOutWhenUnconnected=off
  z_d : Outport  Port=3  VectorParamsAs1DForOutWhenUnconnected=off
  yaw_d : Outport  Port=4  VectorParamsAs1DForOutWhenUnconnected=off
  wires:
  Manual Switch2/1 -> Slider Gain3/1
  Slider Gain3/1 -> yaw_d/1
  Sine Wave2/1 -> Manual Switch2/2
  Constant3/1 -> Manual Switch2/1
  Bus Selector/1 -> MATLAB Function1/5(x)  "<x>"
  MATLAB Function1/2(y_d_) -> y_d/1
  Constant2/1 -> MATLAB Function1/11(z_d_for_land)
  Subsystem/3(zd) -> MATLAB Function1/3(z_d)
  Bus Selector/2 -> MATLAB Function1/6(y)  "<y>"
  Constant1/1 -> MATLAB Function1/10(battery_threshold)
  MATLAB Function1/3(z_d_) -> z_d/1
  droneyeeUAV_states/1 -> Subsystem/2(uavstates), Bus Selector/1
  MATLAB Function1/1(x_d_) -> x_d/1
  Constant4/1 -> MATLAB Function1/12(UAV_NUM)
  Bus Selector/3 -> MATLAB Function1/7(z)  "<z>"
  Constant/1 -> MATLAB Function1/9(sim_time_end)
  Subsystem/1("xd ") -> MATLAB Function1/1(x_d)
  Subsystem/2(yd) -> MATLAB Function1/2(y_d)
  "clock "/1 -> Subsystem/1(clock), MATLAB Function1/4(timestamp)
  droneyeeUAV_bat/1 -> MATLAB Function1/8(battery_status)

== system SIMULINK_U_a_C/CMD_UAV/CMD4 ==
  "clock " : Inport
  droneyeeUAV_states : Inport  Port=2
  droneyeeUAV_bat : Inport  Port=3
  Bus Selector : BusSelector  OutputSignals=x,y,z
  Constant : Constant  Value=sim_end_time
  Constant1 : Constant  Value=battery_threshold
  Constant2 : Constant  Value=z_d_for_land
  Constant3 : Constant  Value=0
  Constant4 : Constant  Value=UAV_NUM
  MATLAB Function1 : MATLAB Function  TreatAsAtomicUnit=on
  Manual Switch2 : ManualSwitch
  Sine Wave2 : Sin  Amplitude=0.3  Frequency=1.0
  Slider Gain3 : simulink/Math Operations/Slider Gain  gain=1  low=0  high=2
  Subsystem : Subsystem
  x_d : Outport  VectorParamsAs1DForOutWhenUnconnected=off
  y_d : Outport  Port=2  VectorParamsAs1DForOutWhenUnconnected=off
  z_d : Outport  Port=3  VectorParamsAs1DForOutWhenUnconnected=off
  yaw_d : Outport  Port=4  VectorParamsAs1DForOutWhenUnconnected=off
  wires:
  Manual Switch2/1 -> Slider Gain3/1
  Slider Gain3/1 -> yaw_d/1
  Sine Wave2/1 -> Manual Switch2/2
  Constant3/1 -> Manual Switch2/1
  Bus Selector/1 -> MATLAB Function1/5(x)  "<x>"
  MATLAB Function1/2(y_d_) -> y_d/1
  Constant2/1 -> MATLAB Function1/11(z_d_for_land)
  Subsystem/3(zd) -> MATLAB Function1/3(z_d)
  Bus Selector/2 -> MATLAB Function1/6(y)  "<y>"
  Constant1/1 -> MATLAB Function1/10(battery_threshold)
  MATLAB Function1/3(z_d_) -> z_d/1
  droneyeeUAV_states/1 -> Subsystem/2(uavstates), Bus Selector/1
  MATLAB Function1/1(x_d_) -> x_d/1
  Constant4/1 -> MATLAB Function1/12(UAV_NUM)
  Bus Selector/3 -> MATLAB Function1/7(z)  "<z>"
  Constant/1 -> MATLAB Function1/9(sim_time_end)
  Subsystem/1("xd ") -> MATLAB Function1/1(x_d)
  Subsystem/2(yd) -> MATLAB Function1/2(y_d)
  "clock "/1 -> Subsystem/1(clock), MATLAB Function1/4(timestamp)
  droneyeeUAV_bat/1 -> MATLAB Function1/8(battery_status)

== system SIMULINK_U_a_C/CMD_UAV/CMD5 ==
  "clock " : Inport
  droneyeeUAV_states : Inport  Port=2
  droneyeeUAV_bat : Inport  Port=3
  Bus Selector : BusSelector  OutputSignals=x,y,z
  Constant : Constant  Value=sim_end_time
  Constant1 : Constant  Value=battery_threshold
  Constant2 : Constant  Value=z_d_for_land
  Constant3 : Constant  Value=0
  Constant4 : Constant  Value=UAV_NUM
  MATLAB Function1 : MATLAB Function  TreatAsAtomicUnit=on
  Manual Switch2 : ManualSwitch
  Sine Wave2 : Sin  Amplitude=0.3  Frequency=1.0
  Slider Gain3 : simulink/Math Operations/Slider Gain  gain=1  low=0  high=2
  Subsystem : Subsystem
  Terminator : Terminator
  x_d : Outport  VectorParamsAs1DForOutWhenUnconnected=off
  y_d : Outport  Port=2  VectorParamsAs1DForOutWhenUnconnected=off
  z_d : Outport  Port=3  VectorParamsAs1DForOutWhenUnconnected=off
  yaw_d : Outport  Port=4  VectorParamsAs1DForOutWhenUnconnected=off
  wires:
  Manual Switch2/1 -> Slider Gain3/1
  Slider Gain3/1 -> yaw_d/1
  Sine Wave2/1 -> Manual Switch2/2
  Constant3/1 -> Manual Switch2/1
  Bus Selector/1 -> MATLAB Function1/5(x)  "<x>"
  MATLAB Function1/2(y_d_) -> y_d/1
  Constant2/1 -> MATLAB Function1/11(z_d_for_land)
  Subsystem/3(zd) -> MATLAB Function1/3(z_d)
  Bus Selector/2 -> MATLAB Function1/6(y)  "<y>"
  Constant1/1 -> MATLAB Function1/10(battery_threshold)
  MATLAB Function1/3(z_d_) -> z_d/1
  MATLAB Function1/1(x_d_) -> x_d/1
  Constant4/1 -> MATLAB Function1/12(UAV_NUM)
  Bus Selector/3 -> MATLAB Function1/7(z)  "<z>"
  Constant/1 -> MATLAB Function1/9(sim_time_end)
  Subsystem/1("xd ") -> MATLAB Function1/1(x_d)
  Subsystem/2(yd) -> MATLAB Function1/2(y_d)
  "clock "/1 -> Subsystem/1(clock), MATLAB Function1/4(timestamp)
  droneyeeUAV_bat/1 -> MATLAB Function1/8(battery_status)
  droneyeeUAV_states/1 -> Subsystem/2(uavstates), Bus Selector/1

== system SIMULINK_U_a_C/CMD_UAV/CMD6 ==
  "clock " : Inport
  droneyeeUAV_states : Inport  Port=2
  droneyeeUAV_bat : Inport  Port=3
  Bus Selector : BusSelector  OutputSignals=x,y,z
  Constant : Constant  Value=sim_end_time
  Constant1 : Constant  Value=battery_threshold
  Constant2 : Constant  Value=z_d_for_land
  Constant3 : Constant  Value=0
  Constant4 : Constant  Value=UAV_NUM
  MATLAB Function1 : MATLAB Function  TreatAsAtomicUnit=on
  Manual Switch2 : ManualSwitch
  Sine Wave2 : Sin  Amplitude=0.3  Frequency=1.0
  Slider Gain3 : simulink/Math Operations/Slider Gain  gain=1  low=0  high=2
  Subsystem : Subsystem
  x_d : Outport  VectorParamsAs1DForOutWhenUnconnected=off
  y_d : Outport  Port=2  VectorParamsAs1DForOutWhenUnconnected=off
  z_d : Outport  Port=3  VectorParamsAs1DForOutWhenUnconnected=off
  yaw_d : Outport  Port=4  VectorParamsAs1DForOutWhenUnconnected=off
  wires:
  Manual Switch2/1 -> Slider Gain3/1
  Slider Gain3/1 -> yaw_d/1
  Sine Wave2/1 -> Manual Switch2/2
  Constant3/1 -> Manual Switch2/1
  MATLAB Function1/2(y_d_) -> y_d/1
  Constant2/1 -> MATLAB Function1/11(z_d_for_land)
  Subsystem/3(zd) -> MATLAB Function1/3(z_d)
  Constant1/1 -> MATLAB Function1/10(battery_threshold)
  MATLAB Function1/3(z_d_) -> z_d/1
  droneyeeUAV_states/1 -> Subsystem/2(uavstates), Bus Selector/1
  MATLAB Function1/1(x_d_) -> x_d/1
  Constant4/1 -> MATLAB Function1/12(UAV_NUM)
  Constant/1 -> MATLAB Function1/9(sim_time_end)
  Subsystem/1("xd ") -> MATLAB Function1/1(x_d)
  Subsystem/2(yd) -> MATLAB Function1/2(y_d)
  "clock "/1 -> Subsystem/1(clock), MATLAB Function1/4(timestamp)
  droneyeeUAV_bat/1 -> MATLAB Function1/8(battery_status)
  Bus Selector/1 -> MATLAB Function1/5(x)  "<x>"
  Bus Selector/2 -> MATLAB Function1/6(y)  "<y>"
  Bus Selector/3 -> MATLAB Function1/7(z)  "<z>"

== system SIMULINK_U_a_C/CMD_UAV/CMD7 ==
  "clock " : Inport
  droneyeeUAV_states : Inport  Port=2
  droneyeeUAV_bat : Inport  Port=3
  Bus Selector : BusSelector  OutputSignals=x,y,z
  Constant : Constant  Value=sim_end_time
  Constant1 : Constant  Value=battery_threshold
  Constant2 : Constant  Value=z_d_for_land
  Constant3 : Constant  Value=0
  Constant4 : Constant  Value=UAV_NUM
  MATLAB Function1 : MATLAB Function  TreatAsAtomicUnit=on
  Manual Switch2 : ManualSwitch
  Sine Wave2 : Sin  Amplitude=0.3  Frequency=1.0
  Slider Gain3 : simulink/Math Operations/Slider Gain  gain=1  low=0  high=2
  Subsystem : Subsystem
  Terminator : Terminator
  x_d : Outport  VectorParamsAs1DForOutWhenUnconnected=off
  y_d : Outport  Port=2  VectorParamsAs1DForOutWhenUnconnected=off
  z_d : Outport  Port=3  VectorParamsAs1DForOutWhenUnconnected=off
  yaw_d : Outport  Port=4  VectorParamsAs1DForOutWhenUnconnected=off
  wires:
  Manual Switch2/1 -> Slider Gain3/1
  Slider Gain3/1 -> yaw_d/1
  Sine Wave2/1 -> Manual Switch2/2
  Constant3/1 -> Manual Switch2/1
  Bus Selector/1 -> MATLAB Function1/5(x)  "<x>"
  MATLAB Function1/2(y_d_) -> y_d/1
  Constant2/1 -> MATLAB Function1/11(z_d_for_land)
  Subsystem/3(zd) -> MATLAB Function1/3(z_d)
  Bus Selector/2 -> MATLAB Function1/6(y)  "<y>"
  Constant1/1 -> MATLAB Function1/10(battery_threshold)
  MATLAB Function1/3(z_d_) -> z_d/1
  MATLAB Function1/1(x_d_) -> x_d/1
  Constant4/1 -> MATLAB Function1/12(UAV_NUM)
  Bus Selector/3 -> MATLAB Function1/7(z)  "<z>"
  Constant/1 -> MATLAB Function1/9(sim_time_end)
  Subsystem/1("xd ") -> MATLAB Function1/1(x_d)
  Subsystem/2(yd) -> MATLAB Function1/2(y_d)
  "clock "/1 -> Subsystem/1(clock), MATLAB Function1/4(timestamp)
  droneyeeUAV_bat/1 -> MATLAB Function1/8(battery_status)
  droneyeeUAV_states/1 -> Subsystem/2(uavstates), Bus Selector/1

== system SIMULINK_U_a_C/CMD_UAV/CMD8 ==
  "clock " : Inport
  droneyeeUAV_states : Inport  Port=2
  droneyeeUAV_bat : Inport  Port=3
  Bus Selector : BusSelector  OutputSignals=x,y,z
  Constant : Constant  Value=sim_end_time
  Constant1 : Constant  Value=battery_threshold
  Constant2 : Constant  Value=z_d_for_land
  Constant3 : Constant  Value=0
  Constant4 : Constant  Value=UAV_NUM
  MATLAB Function1 : MATLAB Function  TreatAsAtomicUnit=on
  Manual Switch2 : ManualSwitch
  Sine Wave2 : Sin  Amplitude=0.3  Frequency=1.0
  Slider Gain3 : simulink/Math Operations/Slider Gain  gain=1  low=0  high=2
  Subsystem : Subsystem
  x_d : Outport  VectorParamsAs1DForOutWhenUnconnected=off
  y_d : Outport  Port=2  VectorParamsAs1DForOutWhenUnconnected=off
  z_d : Outport  Port=3  VectorParamsAs1DForOutWhenUnconnected=off
  yaw_d : Outport  Port=4  VectorParamsAs1DForOutWhenUnconnected=off
  wires:
  Manual Switch2/1 -> Slider Gain3/1
  Slider Gain3/1 -> yaw_d/1
  Sine Wave2/1 -> Manual Switch2/2
  Constant3/1 -> Manual Switch2/1
  MATLAB Function1/2(y_d_) -> y_d/1
  Constant2/1 -> MATLAB Function1/11(z_d_for_land)
  Subsystem/3(zd) -> MATLAB Function1/3(z_d)
  Constant1/1 -> MATLAB Function1/10(battery_threshold)
  MATLAB Function1/3(z_d_) -> z_d/1
  droneyeeUAV_states/1 -> Subsystem/2(uavstates), Bus Selector/1
  MATLAB Function1/1(x_d_) -> x_d/1
  Constant4/1 -> MATLAB Function1/12(UAV_NUM)
  Constant/1 -> MATLAB Function1/9(sim_time_end)
  Subsystem/1("xd ") -> MATLAB Function1/1(x_d)
  Subsystem/2(yd) -> MATLAB Function1/2(y_d)
  "clock "/1 -> Subsystem/1(clock), MATLAB Function1/4(timestamp)
  droneyeeUAV_bat/1 -> MATLAB Function1/8(battery_status)
  Bus Selector/1 -> MATLAB Function1/5(x)  "<x>"
  Bus Selector/2 -> MATLAB Function1/6(y)  "<y>"
  Bus Selector/3 -> MATLAB Function1/7(z)  "<z>"

== system SIMULINK_U_a_C/CMD_UAV/CMD9 ==
  "clock " : Inport
  droneyeeUAV_states : Inport  Port=2
  droneyeeUAV_bat : Inport  Port=3
  Bus Selector : BusSelector  OutputSignals=x,y,z
  Constant : Constant  Value=sim_end_time
  Constant1 : Constant  Value=battery_threshold
  Constant2 : Constant  Value=z_d_for_land
  Constant3 : Constant  Value=0
  Constant4 : Constant  Value=UAV_NUM
  MATLAB Function1 : MATLAB Function  TreatAsAtomicUnit=on
  Manual Switch2 : ManualSwitch
  Sine Wave2 : Sin  Amplitude=0.3  Frequency=1.0
  Slider Gain3 : simulink/Math Operations/Slider Gain  gain=1  low=0  high=2
  Subsystem : Subsystem
  Terminator : Terminator
  x_d : Outport  VectorParamsAs1DForOutWhenUnconnected=off
  y_d : Outport  Port=2  VectorParamsAs1DForOutWhenUnconnected=off
  z_d : Outport  Port=3  VectorParamsAs1DForOutWhenUnconnected=off
  yaw_d : Outport  Port=4  VectorParamsAs1DForOutWhenUnconnected=off
  wires:
  Manual Switch2/1 -> Slider Gain3/1
  Slider Gain3/1 -> yaw_d/1
  Sine Wave2/1 -> Manual Switch2/2
  Constant3/1 -> Manual Switch2/1
  Bus Selector/1 -> MATLAB Function1/5(x)  "<x>"
  MATLAB Function1/2(y_d_) -> y_d/1
  Constant2/1 -> MATLAB Function1/11(z_d_for_land)
  Subsystem/3(zd) -> MATLAB Function1/3(z_d)
  Bus Selector/2 -> MATLAB Function1/6(y)  "<y>"
  Constant1/1 -> MATLAB Function1/10(battery_threshold)
  MATLAB Function1/3(z_d_) -> z_d/1
  MATLAB Function1/1(x_d_) -> x_d/1
  Constant4/1 -> MATLAB Function1/12(UAV_NUM)
  Bus Selector/3 -> MATLAB Function1/7(z)  "<z>"
  Constant/1 -> MATLAB Function1/9(sim_time_end)
  Subsystem/1("xd ") -> MATLAB Function1/1(x_d)
  Subsystem/2(yd) -> MATLAB Function1/2(y_d)
  "clock "/1 -> Subsystem/1(clock), MATLAB Function1/4(timestamp)
  droneyeeUAV_bat/1 -> MATLAB Function1/8(battery_status)
  droneyeeUAV_states/1 -> Subsystem/2(uavstates), Bus Selector/1

== system SIMULINK_U_a_C/CMD_car1/CMD1 ==
  "clock " : Inport
  droneyeeUAV_states : Inport  Port=2
  droneyeeUAV_bat : Inport  Port=3
  Bus Selector : BusSelector  OutputSignals=x,y,z
  Constant : Constant  Value=sim_end_time
  Constant1 : Constant  Value=battery_threshold
  Constant2 : Constant  Value=z_d_for_land
  Constant3 : Constant  Value=0
  Constant4 : Constant  Value=UAV_NUM
  MATLAB Function1 : MATLAB Function  TreatAsAtomicUnit=on
  Manual Switch2 : ManualSwitch
  Sine Wave2 : Sin  Amplitude=0.3  Frequency=1.0
  Slider Gain3 : simulink/Math Operations/Slider Gain  gain=1  low=0  high=2
  Subsystem : Subsystem
  To Workspace : ToWorkspace  VariableName=simout1  SaveFormat=Timeseries  SampleTime=-1
  x_d : Outport  VectorParamsAs1DForOutWhenUnconnected=off
  y_d : Outport  Port=2  VectorParamsAs1DForOutWhenUnconnected=off
  z_d : Outport  Port=3  VectorParamsAs1DForOutWhenUnconnected=off
  yaw_d : Outport  Port=4  VectorParamsAs1DForOutWhenUnconnected=off
  wires:
  Manual Switch2/1 -> Slider Gain3/1
  Slider Gain3/1 -> yaw_d/1
  Sine Wave2/1 -> Manual Switch2/2
  Constant3/1 -> Manual Switch2/1
  MATLAB Function1/2(y_d_) -> y_d/1
  Constant2/1 -> MATLAB Function1/11(z_d_for_land)
  Subsystem/3(zd) -> MATLAB Function1/3(z_d)
  Constant1/1 -> MATLAB Function1/10(battery_threshold)
  MATLAB Function1/3(z_d_) -> z_d/1
  droneyeeUAV_states/1 -> Subsystem/2(uavstates), Bus Selector/1
  MATLAB Function1/1(x_d_) -> To Workspace/1, x_d/1
  Constant4/1 -> MATLAB Function1/12(UAV_NUM)
  Constant/1 -> MATLAB Function1/9(sim_time_end)
  Subsystem/1("xd ") -> MATLAB Function1/1(x_d)
  Subsystem/2(yd) -> MATLAB Function1/2(y_d)
  "clock "/1 -> Subsystem/1(clock), MATLAB Function1/4(timestamp)
  droneyeeUAV_bat/1 -> MATLAB Function1/8(battery_status)
  Bus Selector/1 -> MATLAB Function1/5(x)  "<x>"
  Bus Selector/2 -> MATLAB Function1/6(y)  "<y>"
  Bus Selector/3 -> MATLAB Function1/7(z)  "<z>"

== system SIMULINK_U_a_C/CMD_car1/CMD10 ==
  "clock " : Inport
  droneyeeUAV_states : Inport  Port=2
  droneyeeUAV_bat : Inport  Port=3
  Bus Selector : BusSelector  OutputSignals=x,y,z
  Constant : Constant  Value=sim_end_time
  Constant1 : Constant  Value=battery_threshold
  Constant2 : Constant  Value=z_d_for_land
  Constant3 : Constant  Value=0
  Constant4 : Constant  Value=UAV_NUM
  MATLAB Function1 : MATLAB Function  TreatAsAtomicUnit=on
  Manual Switch2 : ManualSwitch
  Sine Wave2 : Sin  Amplitude=0.3  Frequency=1.0
  Slider Gain3 : simulink/Math Operations/Slider Gain  gain=1  low=0  high=2
  Subsystem : Subsystem
  x_d : Outport  VectorParamsAs1DForOutWhenUnconnected=off
  y_d : Outport  Port=2  VectorParamsAs1DForOutWhenUnconnected=off
  z_d : Outport  Port=3  VectorParamsAs1DForOutWhenUnconnected=off
  yaw_d : Outport  Port=4  VectorParamsAs1DForOutWhenUnconnected=off
  wires:
  Manual Switch2/1 -> Slider Gain3/1
  Slider Gain3/1 -> yaw_d/1
  Sine Wave2/1 -> Manual Switch2/2
  Constant3/1 -> Manual Switch2/1
  MATLAB Function1/2(y_d_) -> y_d/1
  Constant2/1 -> MATLAB Function1/11(z_d_for_land)
  Subsystem/3(zd) -> MATLAB Function1/3(z_d)
  Constant1/1 -> MATLAB Function1/10(battery_threshold)
  MATLAB Function1/3(z_d_) -> z_d/1
  droneyeeUAV_states/1 -> Subsystem/2(uavstates), Bus Selector/1
  MATLAB Function1/1(x_d_) -> x_d/1
  Constant4/1 -> MATLAB Function1/12(UAV_NUM)
  Constant/1 -> MATLAB Function1/9(sim_time_end)
  Subsystem/1("xd ") -> MATLAB Function1/1(x_d)
  Subsystem/2(yd) -> MATLAB Function1/2(y_d)
  "clock "/1 -> Subsystem/1(clock), MATLAB Function1/4(timestamp)
  droneyeeUAV_bat/1 -> MATLAB Function1/8(battery_status)
  Bus Selector/1 -> MATLAB Function1/5(x)  "<x>"
  Bus Selector/2 -> MATLAB Function1/6(y)  "<y>"
  Bus Selector/3 -> MATLAB Function1/7(z)  "<z>"

== system SIMULINK_U_a_C/CMD_car1/CMD2 ==
  "clock " : Inport
  droneyeeUAV_states : Inport  Port=2
  droneyeeUAV_bat : Inport  Port=3
  Bus Selector : BusSelector  OutputSignals=x,y,z
  Constant : Constant  Value=sim_end_time
  Constant1 : Constant  Value=battery_threshold
  Constant2 : Constant  Value=z_d_for_land
  Constant3 : Constant  Value=0
  Constant4 : Constant  Value=UAV_NUM
  MATLAB Function1 : MATLAB Function  TreatAsAtomicUnit=on
  Manual Switch2 : ManualSwitch
  Sine Wave2 : Sin  Amplitude=0.3  Frequency=1.0
  Slider Gain3 : simulink/Math Operations/Slider Gain  gain=1  low=0  high=2
  Subsystem : Subsystem
  x_d : Outport  VectorParamsAs1DForOutWhenUnconnected=off
  y_d : Outport  Port=2  VectorParamsAs1DForOutWhenUnconnected=off
  z_d : Outport  Port=3  VectorParamsAs1DForOutWhenUnconnected=off
  yaw_d : Outport  Port=4  VectorParamsAs1DForOutWhenUnconnected=off
  wires:
  Manual Switch2/1 -> Slider Gain3/1
  Slider Gain3/1 -> yaw_d/1
  Sine Wave2/1 -> Manual Switch2/2
  Constant3/1 -> Manual Switch2/1
  Bus Selector/1 -> MATLAB Function1/5(x)  "<x>"
  MATLAB Function1/2(y_d_) -> y_d/1
  Constant2/1 -> MATLAB Function1/11(z_d_for_land)
  Subsystem/3(zd) -> MATLAB Function1/3(z_d)
  Bus Selector/2 -> MATLAB Function1/6(y)  "<y>"
  Constant1/1 -> MATLAB Function1/10(battery_threshold)
  MATLAB Function1/3(z_d_) -> z_d/1
  droneyeeUAV_states/1 -> Subsystem/2(uavstates), Bus Selector/1
  MATLAB Function1/1(x_d_) -> x_d/1
  Constant4/1 -> MATLAB Function1/12(UAV_NUM)
  Bus Selector/3 -> MATLAB Function1/7(z)  "<z>"
  Constant/1 -> MATLAB Function1/9(sim_time_end)
  Subsystem/1("xd ") -> MATLAB Function1/1(x_d)
  Subsystem/2(yd) -> MATLAB Function1/2(y_d)
  "clock "/1 -> Subsystem/1(clock), MATLAB Function1/4(timestamp)
  droneyeeUAV_bat/1 -> MATLAB Function1/8(battery_status)

== system SIMULINK_U_a_C/CMD_car1/CMD3 ==
  "clock " : Inport
  droneyeeUAV_states : Inport  Port=2
  droneyeeUAV_bat : Inport  Port=3
  Bus Selector : BusSelector  OutputSignals=x,y,z
  Constant : Constant  Value=sim_end_time
  Constant1 : Constant  Value=battery_threshold
  Constant2 : Constant  Value=z_d_for_land
  Constant3 : Constant  Value=0
  Constant4 : Constant  Value=UAV_NUM
  MATLAB Function1 : MATLAB Function  TreatAsAtomicUnit=on
  Manual Switch2 : ManualSwitch
  Sine Wave2 : Sin  Amplitude=0.3  Frequency=1.0
  Slider Gain3 : simulink/Math Operations/Slider Gain  gain=1  low=0  high=2
  Subsystem : Subsystem
  x_d : Outport  VectorParamsAs1DForOutWhenUnconnected=off
  y_d : Outport  Port=2  VectorParamsAs1DForOutWhenUnconnected=off
  z_d : Outport  Port=3  VectorParamsAs1DForOutWhenUnconnected=off
  yaw_d : Outport  Port=4  VectorParamsAs1DForOutWhenUnconnected=off
  wires:
  Manual Switch2/1 -> Slider Gain3/1
  Slider Gain3/1 -> yaw_d/1
  Sine Wave2/1 -> Manual Switch2/2
  Constant3/1 -> Manual Switch2/1
  Bus Selector/1 -> MATLAB Function1/5(x)  "<x>"
  MATLAB Function1/2(y_d_) -> y_d/1
  Constant2/1 -> MATLAB Function1/11(z_d_for_land)
  Subsystem/3(zd) -> MATLAB Function1/3(z_d)
  Bus Selector/2 -> MATLAB Function1/6(y)  "<y>"
  Constant1/1 -> MATLAB Function1/10(battery_threshold)
  MATLAB Function1/3(z_d_) -> z_d/1
  droneyeeUAV_states/1 -> Subsystem/2(uavstates), Bus Selector/1
  MATLAB Function1/1(x_d_) -> x_d/1
  Constant4/1 -> MATLAB Function1/12(UAV_NUM)
  Bus Selector/3 -> MATLAB Function1/7(z)  "<z>"
  Constant/1 -> MATLAB Function1/9(sim_time_end)
  Subsystem/1("xd ") -> MATLAB Function1/1(x_d)
  Subsystem/2(yd) -> MATLAB Function1/2(y_d)
  "clock "/1 -> Subsystem/1(clock), MATLAB Function1/4(timestamp)
  droneyeeUAV_bat/1 -> MATLAB Function1/8(battery_status)

== system SIMULINK_U_a_C/CMD_car1/CMD4 ==
  "clock " : Inport
  droneyeeUAV_states : Inport  Port=2
  droneyeeUAV_bat : Inport  Port=3
  Bus Selector : BusSelector  OutputSignals=x,y,z
  Constant : Constant  Value=sim_end_time
  Constant1 : Constant  Value=battery_threshold
  Constant2 : Constant  Value=z_d_for_land
  Constant3 : Constant  Value=0
  Constant4 : Constant  Value=UAV_NUM
  MATLAB Function1 : MATLAB Function  TreatAsAtomicUnit=on
  Manual Switch2 : ManualSwitch
  Sine Wave2 : Sin  Amplitude=0.3  Frequency=1.0
  Slider Gain3 : simulink/Math Operations/Slider Gain  gain=1  low=0  high=2
  Subsystem : Subsystem
  x_d : Outport  VectorParamsAs1DForOutWhenUnconnected=off
  y_d : Outport  Port=2  VectorParamsAs1DForOutWhenUnconnected=off
  z_d : Outport  Port=3  VectorParamsAs1DForOutWhenUnconnected=off
  yaw_d : Outport  Port=4  VectorParamsAs1DForOutWhenUnconnected=off
  wires:
  Manual Switch2/1 -> Slider Gain3/1
  Slider Gain3/1 -> yaw_d/1
  Sine Wave2/1 -> Manual Switch2/2
  Constant3/1 -> Manual Switch2/1
  Bus Selector/1 -> MATLAB Function1/5(x)  "<x>"
  MATLAB Function1/2(y_d_) -> y_d/1
  Constant2/1 -> MATLAB Function1/11(z_d_for_land)
  Subsystem/3(zd) -> MATLAB Function1/3(z_d)
  Bus Selector/2 -> MATLAB Function1/6(y)  "<y>"
  Constant1/1 -> MATLAB Function1/10(battery_threshold)
  MATLAB Function1/3(z_d_) -> z_d/1
  droneyeeUAV_states/1 -> Subsystem/2(uavstates), Bus Selector/1
  MATLAB Function1/1(x_d_) -> x_d/1
  Constant4/1 -> MATLAB Function1/12(UAV_NUM)
  Bus Selector/3 -> MATLAB Function1/7(z)  "<z>"
  Constant/1 -> MATLAB Function1/9(sim_time_end)
  Subsystem/1("xd ") -> MATLAB Function1/1(x_d)
  Subsystem/2(yd) -> MATLAB Function1/2(y_d)
  "clock "/1 -> Subsystem/1(clock), MATLAB Function1/4(timestamp)
  droneyeeUAV_bat/1 -> MATLAB Function1/8(battery_status)

== system SIMULINK_U_a_C/CMD_car1/CMD5 ==
  "clock " : Inport
  droneyeeUAV_states : Inport  Port=2
  droneyeeUAV_bat : Inport  Port=3
  Bus Selector : BusSelector  OutputSignals=x,y,z
  Constant : Constant  Value=sim_end_time
  Constant1 : Constant  Value=battery_threshold
  Constant2 : Constant  Value=z_d_for_land
  Constant3 : Constant  Value=0
  Constant4 : Constant  Value=UAV_NUM
  MATLAB Function1 : MATLAB Function  TreatAsAtomicUnit=on
  Manual Switch2 : ManualSwitch
  Sine Wave2 : Sin  Amplitude=0.3  Frequency=1.0
  Slider Gain3 : simulink/Math Operations/Slider Gain  gain=1  low=0  high=2
  Subsystem : Subsystem
  Terminator : Terminator
  x_d : Outport  VectorParamsAs1DForOutWhenUnconnected=off
  y_d : Outport  Port=2  VectorParamsAs1DForOutWhenUnconnected=off
  z_d : Outport  Port=3  VectorParamsAs1DForOutWhenUnconnected=off
  yaw_d : Outport  Port=4  VectorParamsAs1DForOutWhenUnconnected=off
  wires:
  Manual Switch2/1 -> Slider Gain3/1
  Slider Gain3/1 -> yaw_d/1
  Sine Wave2/1 -> Manual Switch2/2
  Constant3/1 -> Manual Switch2/1
  Bus Selector/1 -> MATLAB Function1/5(x)  "<x>"
  MATLAB Function1/2(y_d_) -> y_d/1
  Constant2/1 -> MATLAB Function1/11(z_d_for_land)
  Subsystem/3(zd) -> MATLAB Function1/3(z_d)
  Bus Selector/2 -> MATLAB Function1/6(y)  "<y>"
  Constant1/1 -> MATLAB Function1/10(battery_threshold)
  MATLAB Function1/3(z_d_) -> z_d/1
  MATLAB Function1/1(x_d_) -> x_d/1
  Constant4/1 -> MATLAB Function1/12(UAV_NUM)
  Bus Selector/3 -> MATLAB Function1/7(z)  "<z>"
  Constant/1 -> MATLAB Function1/9(sim_time_end)
  Subsystem/1("xd ") -> MATLAB Function1/1(x_d)
  Subsystem/2(yd) -> MATLAB Function1/2(y_d)
  "clock "/1 -> Subsystem/1(clock), MATLAB Function1/4(timestamp)
  droneyeeUAV_bat/1 -> MATLAB Function1/8(battery_status)
  droneyeeUAV_states/1 -> Subsystem/2(uavstates), Bus Selector/1
